simulink model "untitled"  (R2013a)
settings: Solver=ode45  StartTime=0.0  StopTime=10.0  RelTol=1e-3
values from neighbouring files (symbols this model uses):
  czas_skoku = 300    [skrypt.m]
  dTzew = 0    [skrypt.m]
  Tzew = TzewN+i*5    [skrypt.m]
undefined symbols (not defined in the file or in its folder): c, Cva, Cvb, dfw, dPg, fw, g, K, Pg, Ta0, Tb0
settings Model: Creator=Dawidek  LastModifiedBy=Dawidek

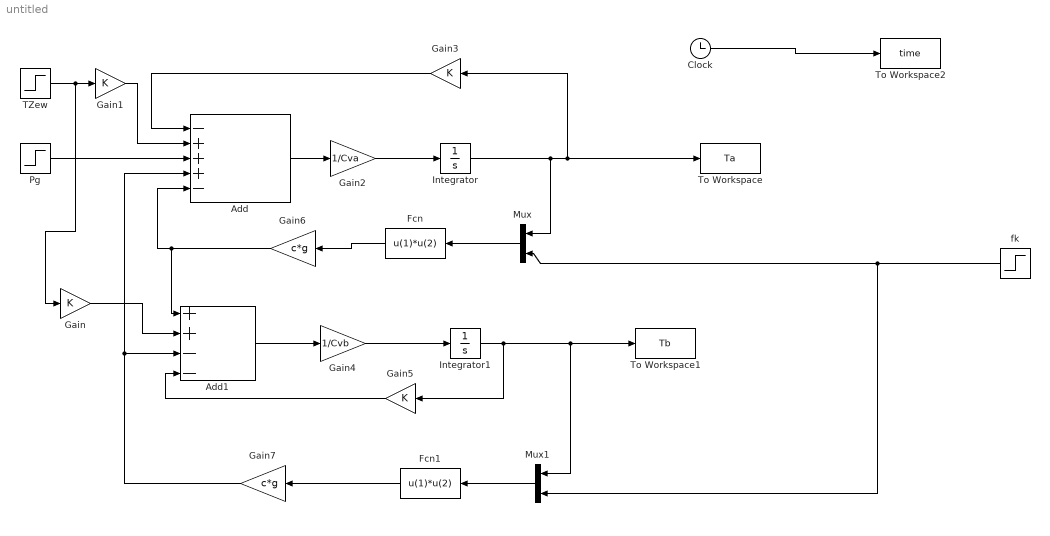
== system untitled ==
  Add : Sum  Inputs=-+++-
  Add1 : Sum  Inputs=++--
  Clock : Clock
  Fcn : Fcn  Expr=u(1)*u(2)
  Fcn1 : Fcn  Expr=u(1)*u(2)
  Gain{,1,3,5} (4 alike) : Gain  Gain=K
  Gain2 : Gain  Gain=1/Cva
  Gain4 : Gain  Gain=1/Cvb
  Gain6 : Gain  Gain=c*g
  Gain7 : Gain  Gain=c*g
  Integrator : Integrator  InitialCondition=Ta0
  Integrator1 : Integrator  InitialCondition=Tb0
  Mux : Mux  Inputs=2
  Mux1 : Mux  Inputs=2
  Pg : Step  Time=czas_skoku  Before=Pg  After=Pg+dPg  SampleTime=0
  TZew : Step  Time=czas_skoku  Before=Tzew  After=Tzew+dTzew  SampleTime=0
  To Workspace : ToWorkspace  VariableName=Ta  SampleTime=-1
  To Workspace1 : ToWorkspace  VariableName=Tb  SampleTime=-1
  To Workspace2 : ToWorkspace  VariableName=time  SampleTime=-1
  fk : Step  Time=czas_skoku  Before=fw  After=fw+dfw  SampleTime=0
  wires:
  TZew/1 -> Gain/1, Gain1/1
  Gain1/1 -> Add/2
  Pg/1 -> Add/3
  Add/1 -> Gain2/1
  Gain2/1 -> Integrator/1
  Integrator/1 -> Mux/1, Gain3/1, To Workspace/1
  Gain3/1 -> Add/1
  fk/1 -> Mux1/2, Mux/2
  Mux/1 -> Fcn/1
  Gain/1 -> Add1/2
  Add1/1 -> Gain4/1
  Gain4/1 -> Integrator1/1
  Integrator1/1 -> Gain5/1, Mux1/1, To Workspace1/1
  Gain5/1 -> Add1/4
  Mux1/1 -> Fcn1/1
  Clock/1 -> To Workspace2/1
  Fcn/1 -> Gain6/1
  Gain6/1 -> Add1/1, Add/5
  Fcn1/1 -> Gain7/1
  Gain7/1 -> Add/4, Add1/3
